simulink model "Tracking_antenna_model"  (R2019b)
settings: Solver=VariableStepAuto  StartTime=0.0  StopTime=simtime  RelTol=1e-3
values from neighbouring files (symbols this model uses):
  Distance = 1    [Tracking_antenna_script.m]
  Gc = 1    [Tracking_antenna_script.m]
  Speed_slope = 0.01    [Tracking_antenna_script.m]
undefined symbols (not defined in the file or in its folder): Selector
libraries: simulink x1
settings Model: Creator=15571272  LastModifiedBy=15571272

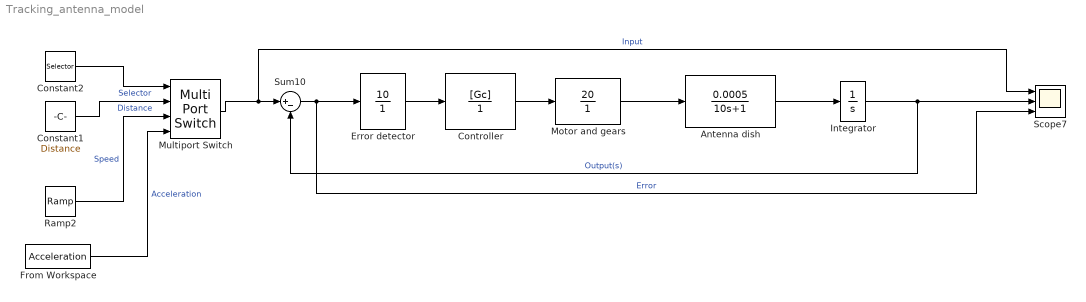
== system Tracking_antenna_model ==
  Antenna dish : TransferFcn  Numerator=[0.0005]  Denominator=[10 1 ]
  Constant1 : Constant  Value=Distance
  Constant2 : Constant  Value=Selector
  Controller : TransferFcn  Numerator=[Gc]  Denominator=[1]
  Error detector : TransferFcn  Numerator=[10]  Denominator=[1]
  From Workspace : FromWorkspace  VariableName=Acceleration  SampleTime=0
  Integrator : Integrator
  Motor and gears : TransferFcn  Numerator=[20]  Denominator=[1]
  Multiport Switch : MultiPortSwitch
  Ramp2 : simulink/Sources/Ramp  slope=Speed_slope  start=0  InitialOutput=0
  Scope7 : Scope  NumInputPorts=3
  Sum10 : Sum  Inputs=|+-
  wires:
  Sum10/1 -> Error detector/1, Scope7/3  "Error"
  Error detector/1 -> Controller/1
  Integrator/1 -> Sum10/2, Scope7/2  "Output(s)"
  Motor and gears/1 -> Antenna dish/1
  Controller/1 -> Motor and gears/1
  Antenna dish/1 -> Integrator/1
  Multiport Switch/1 -> Scope7/1, Sum10/1  "Input"
  Ramp2/1 -> Multiport Switch/3  "Speed"
  Constant2/1 -> Multiport Switch/1  "Selector"
  Constant1/1 -> Multiport Switch/2  "Distance"
  From Workspace/1 -> Multiport Switch/4  "Acceleration"
